simulink model "Ejemplo01_Controladores_servo_ver18"  (R2018b)
settings: Solver=VariableStepAuto  StartTime=0.0  StopTime=2  RelTol=1e-3
values from neighbouring files (symbols this model uses):
  B = 0.003026    [MotorDC.m]
  J = 0.00246    [MotorDC.m]
  Ka = 0.25    [MotorDC.m]
  Km = 0.25    [MotorDC.m]
  L = 0.0047    [MotorDC.m]
  R = 2.27    [MotorDC.m]
  Ti = 0.1    [MotorDC.m]
undefined symbols (not defined in the file or in its folder): Td
settings Model: Creator=cjuar  LastModifiedBy=cjuar
settings DataIOCC: ReturnWorkspaceOutputs=on
settings DebuggingCC: UnconnectedInputMsg=none  UnconnectedOutputMsg=none  UnconnectedLineMsg=none
settings ModelReferenceCC: EnableRefExpFcnMdlSchedulingChecks=off
settings RTWCC: Description=Generic Real-Time Target
settings ConfigComp: CovBoundaryAbsTol=1.0e-5

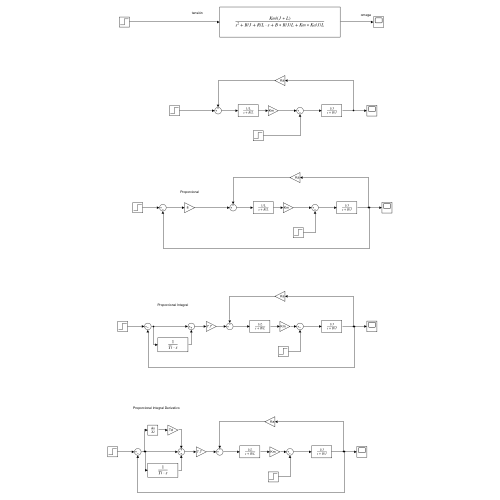
[thumbnail: Simulink's stored preview of the top-level diagram]
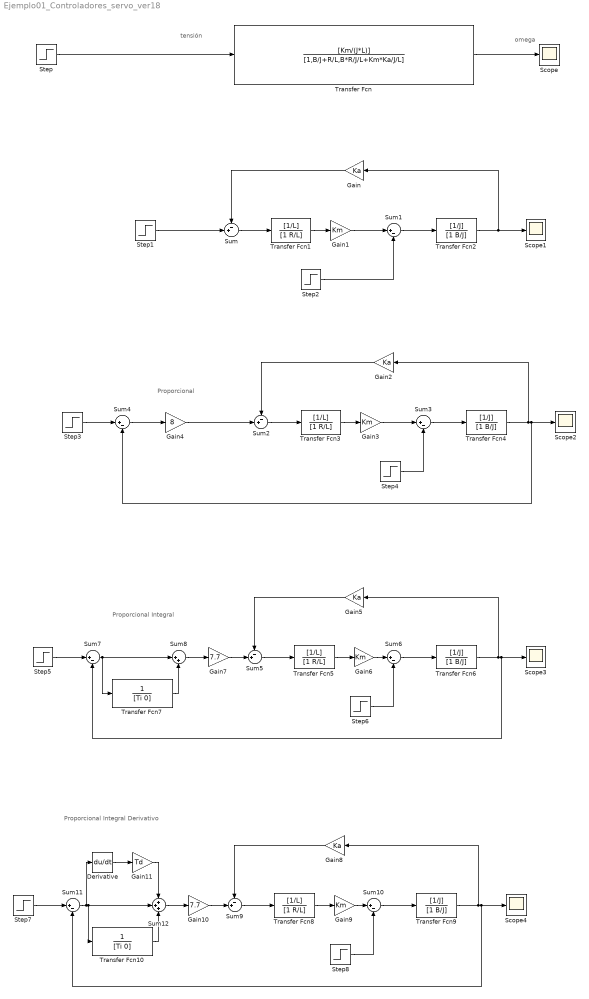
== system Ejemplo01_Controladores_servo_ver18 ==
  note: Proporcional
  note: tensión
  note: omega
  note: Proporcional Integral
  note: Proporcional Integral Derivativo
  Derivative : Derivative
  Gain{,2,5,8} (4 alike) : Gain  Gain=Ka
  Gain{1,3,6,9} (4 alike) : Gain  Gain=Km
  Gain10 : Gain  Gain=7.7
  Gain11 : Gain  Gain=Td
  Gain4 : Gain  Gain=8
  Gain7 : Gain  Gain=7.7
  Scope{,1..4} (5 alike) : Scope
  Step : Step  SampleTime=0
  Step1 : Step  SampleTime=0
  Step2 : Step  After=0  SampleTime=0
  Step3 : Step  After=3.5  SampleTime=0
  Step4 : Step  Time=1.2  After=0.1  SampleTime=0
  Step5 : Step  After=3.5  SampleTime=0
  Step6 : Step  Time=1.2  After=0.1  SampleTime=0
  Step7 : Step  After=3.5  SampleTime=0
  Step8 : Step  Time=1.2  After=0.1  SampleTime=0
  Sum{,2,5,9} (4 alike) : Sum  Inputs=-+|
  Sum{1,3..4,6..7,10..11} (7 alike) : Sum  Inputs=|+-
  Sum12 : Sum  Inputs=+++
  Sum8 : Sum  Inputs=|++
  Transfer Fcn : TransferFcn  Numerator=[Km/(J*L)]  Denominator=[1,B/J+R/L,B*R/J/L+Km*Ka/J/L]
  Transfer Fcn{1,3,5,8} (4 alike) : TransferFcn  Numerator=[1/L]  Denominator=[1 R/L]
  Transfer Fcn10 : TransferFcn  Denominator=[Ti 0]
  Transfer Fcn{2,4,6,9} (4 alike) : TransferFcn  Numerator=[1/J]  Denominator=[1 B/J]
  Transfer Fcn7 : TransferFcn  Denominator=[Ti 0]
  wires:
  Step/1 -> Transfer Fcn/1
  Transfer Fcn/1 -> Scope/1
  Sum/1 -> Transfer Fcn1/1
  Transfer Fcn1/1 -> Gain1/1
  Gain1/1 -> Sum1/1
  Sum1/1 -> Transfer Fcn2/1
  Transfer Fcn2/1 -> Gain/1, Scope1/1
  Step1/1 -> Sum/2
  Gain/1 -> Sum/1
  Step2/1 -> Sum1/2
  Sum3/1 -> Transfer Fcn4/1
  Transfer Fcn4/1 -> Gain2/1, Scope2/1, Sum4/2
  Sum2/1 -> Transfer Fcn3/1
  Transfer Fcn3/1 -> Gain3/1
  Gain2/1 -> Sum2/1
  Gain3/1 -> Sum3/1
  Step4/1 -> Sum3/2
  Gain4/1 -> Sum2/2
  Step3/1 -> Sum4/1
  Sum4/1 -> Gain4/1
  Step5/1 -> Sum7/1
  Step6/1 -> Sum6/2
  Transfer Fcn5/1 -> Gain6/1
  Gain5/1 -> Sum5/1
  Sum5/1 -> Transfer Fcn5/1
  Gain6/1 -> Sum6/1
  Sum6/1 -> Transfer Fcn6/1
  Transfer Fcn6/1 -> Gain5/1, Scope3/1, Sum7/2
  Gain7/1 -> Sum5/2
  Sum7/1 -> Sum8/1, Transfer Fcn7/1
  Sum8/1 -> Gain7/1
  Transfer Fcn7/1 -> Sum8/2
  Gain10/1 -> Sum9/2
  Transfer Fcn9/1 -> Gain8/1, Scope4/1, Sum11/2
  Transfer Fcn8/1 -> Gain9/1
  Step7/1 -> Sum11/1
  Sum12/1 -> Gain10/1
  Gain8/1 -> Sum9/1
  Sum10/1 -> Transfer Fcn9/1
  Sum9/1 -> Transfer Fcn8/1
  Gain9/1 -> Sum10/1
  Sum11/1 -> Derivative/1, Sum12/2, Transfer Fcn10/1
  Step8/1 -> Sum10/2
  Derivative/1 -> Gain11/1
  Gain11/1 -> Sum12/1
  Transfer Fcn10/1 -> Sum12/3
